simulink model "boost_simulink"  (R2021a)
settings: Solver=FixedStepDiscrete  StartTime=0.0  StopTime=0.5  FixedStep=sampleTime  MaxStep=1e-4  RelTol=1e-4  EnableMultiTasking=on
InitFcn:
  | boost_parameters
model workspace (MAT data in the model file):
  Phase1 = 0
values from neighbouring files (symbols this model uses):
  CoutModulesp = 271e-6    (= 0.000271)    [boost_parameters.m]    (also in unbalance_boost.m)
  CoutModuless = 544e-6    (= 0.000544)    [boost_parameters.m]
  D = (1-Vin/Vout)    (= 0.4)    [boost_parameters.m]    (also in calculations.m = (1-VinOneModule/VoutOneModule); flying_capacitor_parameters.m = 0.25; unbalance_boost.m = 0.25)
  Lcoilsp = 0.517e-3    (= 0.000517)    [boost_parameters.m]    (also in unbalance_boost.m = 0.001034)
  Lcoilss = 0.129e-3    (= 0.000129)    [boost_parameters.m]
  ModuleAPhase = 0    [boost_parameters.m]    (also in flying_capacitor_parameters.m = 90; unbalance_boost.m)
  ModuleBPhase = 180    [boost_parameters.m]    (also in flying_capacitor_parameters.m = 270; unbalance_boost.m = 90)
  ModuleCPhase = 180    [boost_parameters.m]    (also in flying_capacitor_parameters.m = 0)
  ModuleDPhase = 0    [boost_parameters.m]    (also in flying_capacitor_parameters.m = 180)
  Rcoil = 1e-3    (= 0.001)    [boost_parameters.m]    (also in unbalance_boost.m)
  sampleTime = 5e-8    (= 5e-08)    [boost_parameters.m]    (also in flying_capacitor_parameters.m = 5e-07; unbalance_boost.m)
  Vin = 900    [boost_parameters.m]    (also in flying_capacitor_parameters.m; main.m = 880; unbalance_boost.m)
libraries: spsSeriesRLCBranchLib x19, spsVoltageMeasurementLib x19, spsCurrentMeasurementLib x13, spsDiodeLib x8, spsIGBTDiodeLib x8, simulink x8, spsTriangleGeneratorLib x4, spsDCVoltageSourceLib x2, spspowerguiLib x1
settings Model: Creator=The MathWorks, Inc.  LastModifiedBy=enes_
settings SolverCC: AlgebraicLoopSolver=TrustRegion  SolverResetMethod=Robust
settings OptimizationCC: EfficientFloat2IntCast=on  LifeSpan=inf
settings DebuggingCC: ReadBeforeWriteMsg=DisableAll  WriteAfterWriteMsg=DisableAll  WriteAfterReadMsg=DisableAll  UniqueDataStoreMsg=error  StrictBusMsg=ErrorOnBusTreatedAsVector  SFUnexpectedBacktrackingDiag=warning  SFNoUnconditionalDefaultTransitionDiag=warning  SFExecutionAtInitializationDiag=none  SFMachineParentedDataDiag=warning  ArithmeticOperatorsInVariantConditions=warning
settings ModelReferenceCC: UpdateModelReferenceTargets=IfOutOfDate
settings SFSimCC: SFSimEcho=off  SimUseLocalCustomCode=off  CustomCodeUndefinedFunction=UseInterfaceOnly
settings RTWCC: RTWUseLocalCustomCode=off
settings CodeAppCC: StateflowObjectComments=on
settings GRTTargetCC: TargetLangStandard=C89/C90 (ANSI)
settings ConfigComp: CovMetricSettings=dw  CovSaveCumulativeToWorkspaceVar=on  CovSaveSingleToWorkspaceVar=on  CovExternalEMLEnable=off
settings SimscapeCC: SimscapeNormalizeSystem=off  SimscapeNominalValues={1, 'bar'; 1, 'cm^3/s'; 1, 'bar*kg/s'; 1, 'kJ/kg'; 1, 'kW'; }

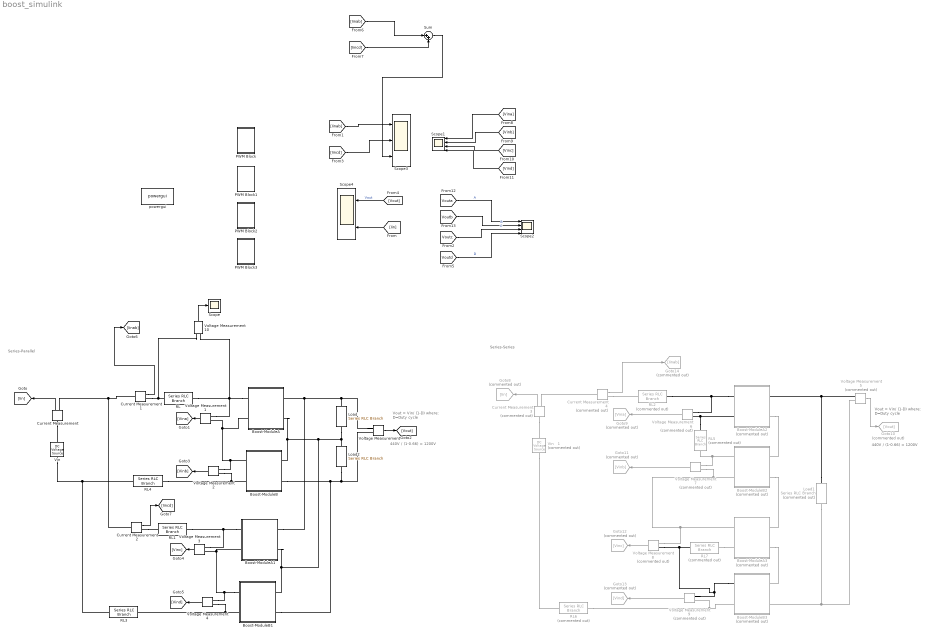
== system boost_simulink ==
  note: Series-Parallel
  note: Vout = Vin/ (1-D)
      | where: D=Duty cycle
  note: 440V / (1-0.66) = 1200V
  note: Series-Series
  note: 440V / (1-0.66) = 1200V
  note: Vout = Vin/ (1-D)
      | where: D=Duty cycle
  Boost-ModuleA : Subsystem
  Boost-ModuleA1 : Subsystem
  Boost-ModuleA2 : Subsystem  Commented=on
  Boost-ModuleA3 : Subsystem  Commented=on
  Boost-ModuleB : Subsystem
  Boost-ModuleB1 : Subsystem
  Boost-ModuleB2 : Subsystem  Commented=on
  Boost-ModuleB3 : Subsystem  Commented=on
  Current Measurement : spsCurrentMeasurementLib/Current Measurement  PhasorSimulation=off  OutputType=Complex  PSBequivalent=0
  Current Measurement1 : spsCurrentMeasurementLib/Current Measurement  PhasorSimulation=off  OutputType=Complex  PSBequivalent=0
  Current Measurement2 : spsCurrentMeasurementLib/Current Measurement  PhasorSimulation=off  OutputType=Complex  PSBequivalent=0
  Current Measurement3 : spsCurrentMeasurementLib/Current Measurement  Commented=on  PhasorSimulation=off  OutputType=Complex  PSBequivalent=0
  Current Measurement4 : spsCurrentMeasurementLib/Current Measurement  Commented=on  PhasorSimulation=off  OutputType=Complex  PSBequivalent=0
  Goto10 : Goto  Commented=on  GotoTag=Vout
  Goto11 : Goto  Commented=on  GotoTag=Vinb
  Goto12 : Goto  Commented=on  GotoTag=Vinc
  Goto13 : Goto  Commented=on  GotoTag=Vind
  Goto14 : Goto  Commented=on  GotoTag=Iinab
  Goto8 : Goto  Commented=on  GotoTag=Iin
  Goto9 : Goto  Commented=on  GotoTag=Vina
  Load : spsSeriesRLCBranchLib/Series RLC Branch  LConnTagsString=__new0  RConnTagsString=__new0  BranchType=R  Resistance=36  Inductance=200e-6  SetiL0=off  InitialCurrent=0  Capacitance=400e-6  Setx0=off  InitialVoltage=0  Measurements=None
  Load1 : spsSeriesRLCBranchLib/Series RLC Branch  Commented=on  LConnTagsString=__new0  RConnTagsString=__new0  BranchType=R  Resistance=72  Inductance=200e-6  SetiL0=off  InitialCurrent=0  Capacitance=400e-6  Setx0=off  InitialVoltage=0  Measurements=None
  Load2 : spsSeriesRLCBranchLib/Series RLC Branch  LConnTagsString=__new0  RConnTagsString=__new0  BranchType=R  Resistance=36  Inductance=200e-6  SetiL0=off  InitialCurrent=0  Capacitance=400e-6  Setx0=off  InitialVoltage=0  Measurements=None
  PWM Block : Subsystem
  PWM Block1 : Subsystem
  PWM Block2 : Subsystem
  PWM Block3 : Subsystem
  RL{,1,3..4} (4 alike) : spsSeriesRLCBranchLib/Series RLC Branch  LConnTagsString=__new0  RConnTagsString=__new0  BranchType=L  Resistance=Rcoil  Inductance=Lcoilsp  SetiL0=off  InitialCurrent=8  Capacitance=1e-6  Setx0=off  InitialVoltage=0  Measurements=None
  RL{2,5..7} (4 alike) : spsSeriesRLCBranchLib/Series RLC Branch  Commented=on  LConnTagsString=__new0  RConnTagsString=__new0  BranchType=L  Resistance=Rcoil  Inductance=Lcoilss  SetiL0=off  InitialCurrent=8  Capacitance=1e-6  Setx0=off  InitialVoltage=0  Measurements=None
  Scope : Scope
  Scope1 : Scope  NumInputPorts=4
  Scope2 : Scope  NumInputPorts=4
  Scope3 : Scope  NumInputPorts=3
  Scope4 : Scope  NumInputPorts=2
  Sum : Sum  Inputs=|++
  "Vin   " : spsDCVoltageSourceLib/DC Voltage Source  Amplitude=Vin  Measurements=None
  Vin   1 : spsDCVoltageSourceLib/DC Voltage Source  Commented=on  Amplitude=Vin  Measurements=None
  Voltage Measurement{,1..4,10} (6 alike) : spsVoltageMeasurementLib/Voltage Measurement  PhasorSimulation=off  OutputType=Complex  PSBequivalent=0
  Voltage Measurement{5..9} (5 alike) : spsVoltageMeasurementLib/Voltage Measurement  Commented=on  PhasorSimulation=off  OutputType=Complex  PSBequivalent=0
  powergui : spspowerguiLib/powergui  Priority=1  SimulationMode=Discrete  SampleTime=sampleTime  frequency=60  Iterations=50  frequencyindice=0  Pbase=100e6  ErrMax=1e-4  UnitsV=kV  UnitsW=MW  buscounter=0  FunctionMessages=off  echomessages=off  EnableUseOfTLC=off  CurrentSourceSwitches=off  DisableSnubberDevices=off  DisableRonSwitches=off  DisableVfSwitches=off  DisplayEquations=off  AutomaticDiscreteSolvers=off  SolverType=Tustin/Backward Euler (TBE)  Interpol=off  ExternalGateDelay=off  methode=off  Ts=100  x0status=blocks  SPID=on  SwTol=0  HookPort=off  NonlinearTolerance=1e-4  nMaxIteration=100  ContinueOnMaxIteration=off  RestoreLinks=warning  ResistiveCurrentMeasurement=off  Frange=[0:2:500]  Ylog=off  Xlog=on  ShowGrid=off  save=off  variable=ZData  structure=0  ZoomFFT=off  StartTime=0.0  cycles=1  DisplayStyle=1  fundamental=60  FreqAxis=off  MaxFrequency=1000  frequencyindicesteady=1  RmsSteady=1  display=off
  wires:
  [Vout] -> Scope4/1  "Vout"
  [Iin] -> Scope4/2
  [Vina] -> Scope1/1
  [Vinb] -> Scope1/2
  [Vinc] -> Scope1/3
  [Vind] -> Scope1/4
  [Iincd] -> Scope3/2
  [Iinab] -> Scope3/1
  [Vouta] -> Scope2/1  "A"
  [Voutb] -> Scope2/2  "B"
  [Voutc] -> Scope2/3  "C"
  [Voutd] -> Scope2/4  "D"
  Current Measurement2/1 -> [Iincd]
  Current Measurement1/1 -> [Iinab]
  Voltage Measurement2/1 -> [Vinb]
  Voltage Measurement4/1 -> [Vind]
  Voltage Measurement3/1 -> [Vinc]
  Voltage Measurement1/1 -> [Vina]
  Current Measurement/1 -> [Iin]
  Voltage Measurement/1 -> [Vout]
  Current Measurement4/1 -> Goto14/1
  Voltage Measurement7/1 -> Goto11/1
  Voltage Measurement9/1 -> Goto13/1
  Voltage Measurement8/1 -> Goto12/1
  Current Measurement3/1 -> Goto8/1
  Voltage Measurement5/1 -> Goto10/1
  Voltage Measurement6/1 -> Goto9/1
  [Iincd] -> Sum/2
  [Iinab] -> Sum/1
  Sum/1 -> Scope3/3
  Voltage Measurement10/1 -> Scope/1
  connections:
  Current Measurement2/RConn1 -- RL1/LConn1
  Current Measurement1/RConn1 -- Voltage Measurement10/LConn1 -- RL/LConn1
  Boost-ModuleA/LConn1 -- RL/RConn1 -- Voltage Measurement10/LConn2 -- Voltage Measurement1/LConn1
  Boost-ModuleA1/LConn1 -- RL1/RConn1 -- Voltage Measurement3/LConn1
  Current Measurement1/LConn1 -- Current Measurement2/LConn1 -- Current Measurement/RConn1
  Boost-ModuleB/RConn2 -- Boost-ModuleB1/RConn2 -- Load2/RConn1 -- Voltage Measurement/LConn2
  Boost-ModuleA/LConn2 -- Voltage Measurement2/LConn1 -- Boost-ModuleB/LConn1 -- Voltage Measurement1/LConn2
  Boost-ModuleB1/LConn1 -- Boost-ModuleA1/LConn2 -- Voltage Measurement3/LConn2 -- Voltage Measurement4/LConn1
  Voltage Measurement2/LConn2 -- RL4/RConn1 -- Boost-ModuleB/LConn2
  Voltage Measurement/LConn1 -- Load/LConn1 -- Boost-ModuleA1/RConn1 -- Boost-ModuleA/RConn1
  Current Measurement/LConn1 -- "Vin   "/RConn1
  RL5/LConn1 -- Boost-ModuleA2/LConn2 -- Voltage Measurement6/LConn2
  Boost-ModuleA2/LConn1 -- RL2/RConn1 -- Voltage Measurement6/LConn1
  Load1/RConn1 -- Voltage Measurement5/LConn2 -- Boost-ModuleB3/RConn2
  Boost-ModuleB2/LConn2 -- Voltage Measurement7/LConn2 -- Boost-ModuleA3/LConn1 -- Voltage Measurement8/LConn1
  Current Measurement4/LConn1 -- Current Measurement3/RConn1
  Boost-ModuleB3/LConn1 -- RL7/LConn1 -- Voltage Measurement8/LConn2 -- Voltage Measurement9/LConn1
  Load1/LConn1 -- Voltage Measurement5/LConn1 -- Boost-ModuleA2/RConn1
  Boost-ModuleA2/RConn2 -- Boost-ModuleB2/RConn1
  Current Measurement3/LConn1 -- Vin   1/RConn1
  Current Measurement4/RConn1 -- RL2/LConn1
  Boost-ModuleA3/RConn2 -- Boost-ModuleB3/RConn1
  Boost-ModuleB3/LConn2 -- RL6/RConn1 -- Voltage Measurement9/LConn2
  Boost-ModuleB2/RConn2 -- Boost-ModuleA3/RConn1
  Boost-ModuleB1/LConn2 -- Voltage Measurement4/LConn2 -- RL3/RConn1
  RL3/LConn1 -- "Vin   "/LConn1 -- RL4/LConn1
  RL5/RConn1 -- Boost-ModuleB2/LConn1 -- Voltage Measurement7/LConn1
  Vin   1/LConn1 -- RL6/LConn1
  RL7/RConn1 -- Boost-ModuleA3/LConn2
  Boost-ModuleA1/RConn2 -- Boost-ModuleB/RConn1 -- Boost-ModuleA/RConn2 -- Load/RConn1 -- Load2/LConn1 -- Boost-ModuleB1/RConn1

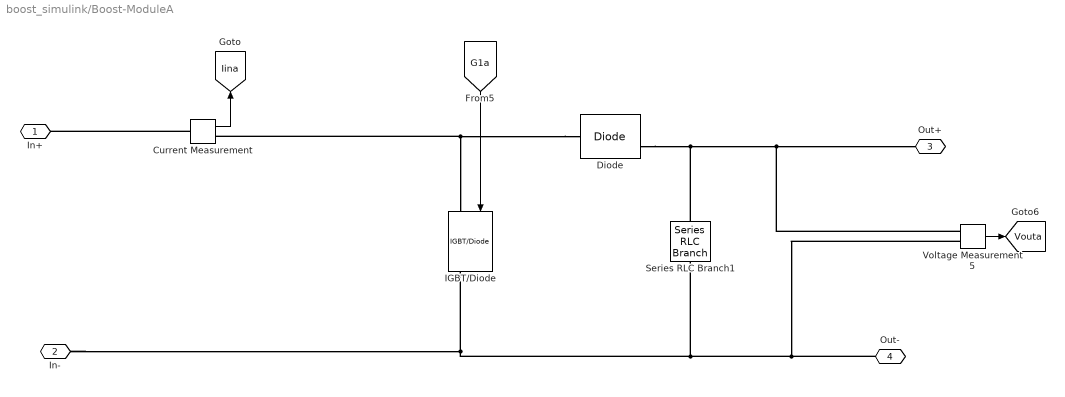
== system boost_simulink/Boost-ModuleA ==
  Current Measurement : spsCurrentMeasurementLib/Current Measurement  PhasorSimulation=off  OutputType=Complex  PSBequivalent=0
  Diode : spsDiodeLib/Diode  Ron=0.001  Lon=0  Vf=0.8  IC=0  UseSnubber=0  Rs=500  Cs=250e-9  Measurements=on
  IGBT/Diode : spsIGBTDiodeLib/IGBT//Diode  Ron=1e-3  Rs=1e5  Cs=inf  Measurements=on
  Series RLC Branch1 : spsSeriesRLCBranchLib/Series RLC Branch  LConnTagsString=__new0  RConnTagsString=__new0  BranchType=C  Resistance=1e-4  Inductance=200e-6  SetiL0=off  InitialCurrent=0  Capacitance=CoutModulesp  Setx0=off  InitialVoltage=1200  Measurements=None
  Voltage Measurement5 : spsVoltageMeasurementLib/Voltage Measurement  PhasorSimulation=off  OutputType=Complex  PSBequivalent=0
  In+ : PMIOPort  Side=Left
  In- : PMIOPort  Port=2  Side=Left
  Out+ : PMIOPort  Port=3  Side=Right
  Out- : PMIOPort  Port=4  Side=Right
  tag scope: Iina=global, Vouta=global
  wires:
  [G1a] -> IGBT/Diode/1
  Current Measurement/1 -> [Iina]
  Voltage Measurement5/1 -> [Vouta]
  connections:
  Diode/LConn1 -- IGBT/Diode/LConn1 -- Current Measurement/RConn1
  Series RLC Branch1/LConn1 -- Diode/RConn1 -- Voltage Measurement5/LConn1 -- Out+/RConn1
  Current Measurement/LConn1 -- In+/RConn1
  Out-/RConn1 -- Voltage Measurement5/LConn2 -- In-/RConn1 -- IGBT/Diode/RConn1 -- Series RLC Branch1/RConn1

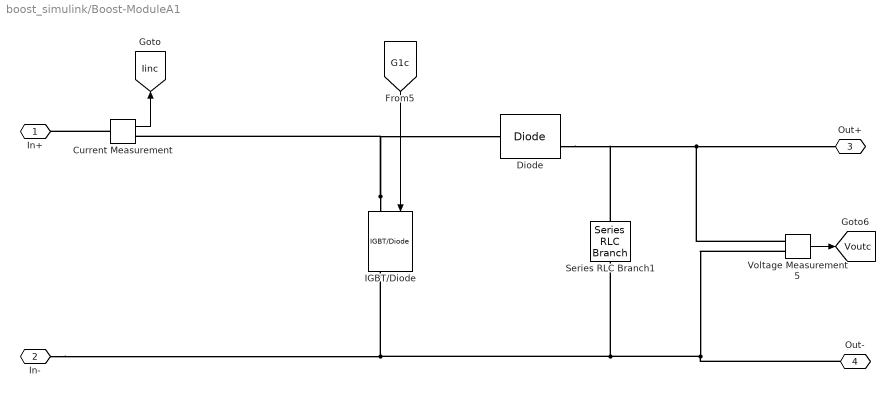
== system boost_simulink/Boost-ModuleA1 ==
  Current Measurement : spsCurrentMeasurementLib/Current Measurement  PhasorSimulation=off  OutputType=Complex  PSBequivalent=0
  Diode : spsDiodeLib/Diode  Ron=0.001  Lon=0  Vf=0.8  IC=0  UseSnubber=0  Rs=500  Cs=250e-9  Measurements=on
  IGBT/Diode : spsIGBTDiodeLib/IGBT//Diode  Ron=1e-3  Rs=1e5  Cs=inf  Measurements=on
  Series RLC Branch1 : spsSeriesRLCBranchLib/Series RLC Branch  LConnTagsString=__new0  RConnTagsString=__new0  BranchType=C  Resistance=1e-4  Inductance=200e-6  SetiL0=off  InitialCurrent=0  Capacitance=CoutModulesp  Setx0=off  InitialVoltage=1200  Measurements=None
  Voltage Measurement5 : spsVoltageMeasurementLib/Voltage Measurement  PhasorSimulation=off  OutputType=Complex  PSBequivalent=0
  In+ : PMIOPort  Side=Left
  In- : PMIOPort  Port=2  Side=Left
  Out+ : PMIOPort  Port=3  Side=Right
  Out- : PMIOPort  Port=4  Side=Right
  tag scope: Iinc=global, Voutc=global
  wires:
  [G1c] -> IGBT/Diode/1
  Current Measurement/1 -> [Iinc]
  Voltage Measurement5/1 -> [Voutc]
  connections:
  IGBT/Diode/LConn1 -- Diode/LConn1 -- Current Measurement/RConn1
  Voltage Measurement5/LConn1 -- Out+/RConn1 -- Series RLC Branch1/LConn1 -- Diode/RConn1
  Current Measurement/LConn1 -- In+/RConn1
  Voltage Measurement5/LConn2 -- Out-/RConn1 -- Series RLC Branch1/RConn1 -- In-/RConn1 -- IGBT/Diode/RConn1

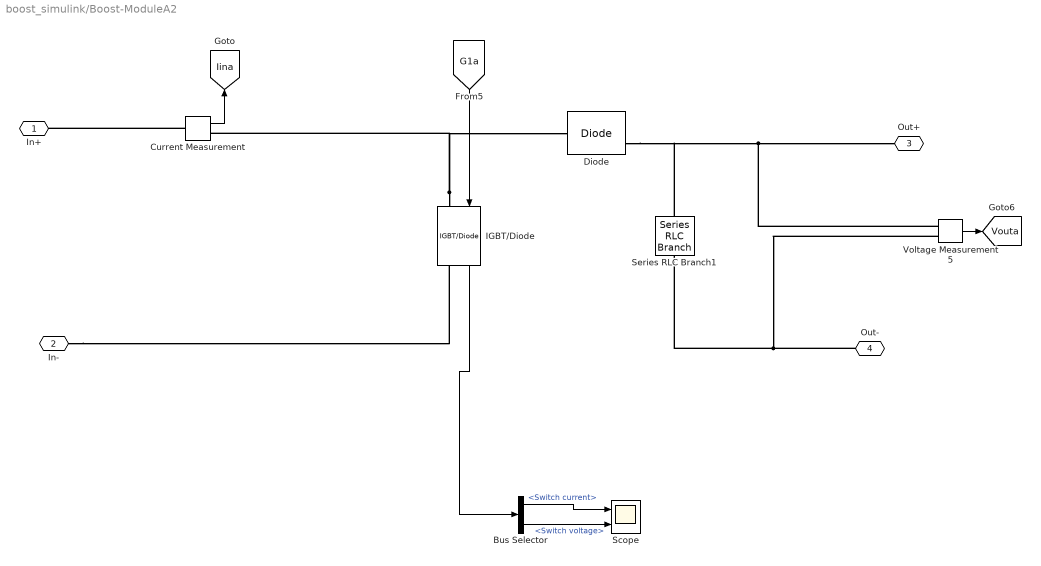
== system boost_simulink/Boost-ModuleA2 ==
  Bus Selector : BusSelector  OutputSignals=Switch current,Switch voltage
  Current Measurement : spsCurrentMeasurementLib/Current Measurement  PhasorSimulation=off  OutputType=Complex  PSBequivalent=0
  Diode : spsDiodeLib/Diode  Ron=0.001  Lon=0  Vf=0.8  IC=0  UseSnubber=0  Rs=500  Cs=250e-9  Measurements=on
  IGBT/Diode : spsIGBTDiodeLib/IGBT//Diode  Ron=1e-3  Rs=1e5  Cs=inf  Measurements=on
  Scope : Scope  NumInputPorts=2
  Series RLC Branch1 : spsSeriesRLCBranchLib/Series RLC Branch  LConnTagsString=__new0  RConnTagsString=__new0  BranchType=C  Resistance=1e-4  Inductance=200e-6  SetiL0=off  InitialCurrent=0  Capacitance=CoutModuless  Setx0=off  InitialVoltage=1200  Measurements=None
  Voltage Measurement5 : spsVoltageMeasurementLib/Voltage Measurement  PhasorSimulation=off  OutputType=Complex  PSBequivalent=0
  In+ : PMIOPort  Side=Left
  In- : PMIOPort  Port=2  Side=Left
  Out+ : PMIOPort  Port=3  Side=Right
  Out- : PMIOPort  Port=4  Side=Right
  tag scope: Iina=global, Vouta=global
  wires:
  [G1a] -> IGBT/Diode/1
  Current Measurement/1 -> [Iina]
  Voltage Measurement5/1 -> [Vouta]
  IGBT/Diode/1 -> Bus Selector/1
  Bus Selector/1 -> Scope/1  "<Switch current>"
  Bus Selector/2 -> Scope/2  "<Switch voltage>"
  connections:
  IGBT/Diode/LConn1 -- Diode/LConn1 -- Current Measurement/RConn1
  Voltage Measurement5/LConn1 -- Out+/RConn1 -- Series RLC Branch1/LConn1 -- Diode/RConn1
  Current Measurement/LConn1 -- In+/RConn1
  In-/RConn1 -- IGBT/Diode/RConn1
  Out-/RConn1 -- Series RLC Branch1/RConn1 -- Voltage Measurement5/LConn2

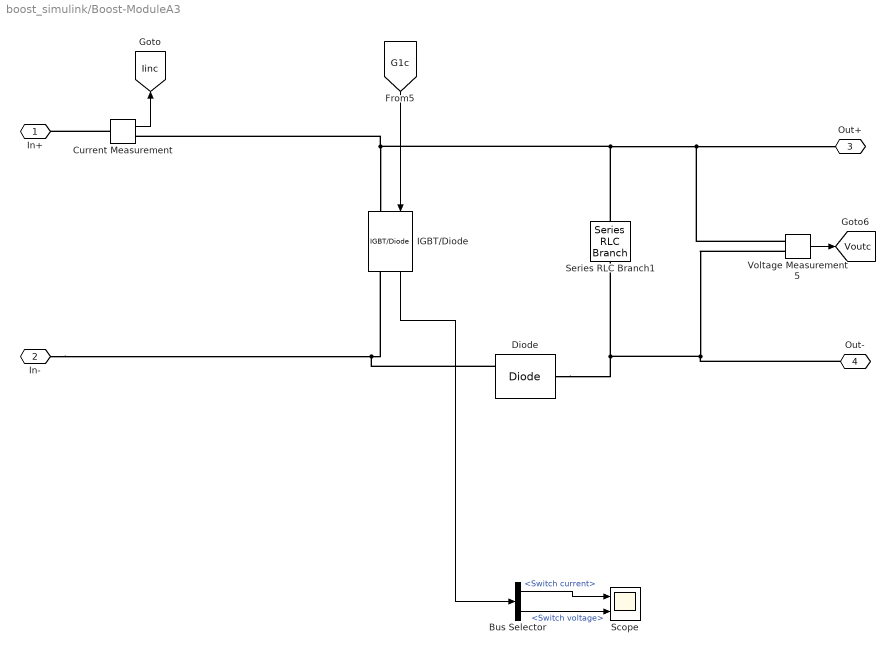
== system boost_simulink/Boost-ModuleA3 ==
  Bus Selector : BusSelector  OutputSignals=Switch current,Switch voltage
  Current Measurement : spsCurrentMeasurementLib/Current Measurement  PhasorSimulation=off  OutputType=Complex  PSBequivalent=0
  Diode : spsDiodeLib/Diode  Ron=0.001  Lon=0  Vf=0.8  IC=0  UseSnubber=0  Rs=500  Cs=250e-9  Measurements=on
  IGBT/Diode : spsIGBTDiodeLib/IGBT//Diode  Ron=1e-3  Rs=1e5  Cs=inf  Measurements=on
  Scope : Scope  NumInputPorts=2
  Series RLC Branch1 : spsSeriesRLCBranchLib/Series RLC Branch  LConnTagsString=__new0  RConnTagsString=__new0  BranchType=C  Resistance=1e-4  Inductance=200e-6  SetiL0=off  InitialCurrent=0  Capacitance=CoutModuless  Setx0=off  InitialVoltage=1200  Measurements=None
  Voltage Measurement5 : spsVoltageMeasurementLib/Voltage Measurement  PhasorSimulation=off  OutputType=Complex  PSBequivalent=0
  In+ : PMIOPort  Side=Left
  In- : PMIOPort  Port=2  Side=Left
  Out+ : PMIOPort  Port=3  Side=Right
  Out- : PMIOPort  Port=4  Side=Right
  tag scope: Iinc=global, Voutc=global
  wires:
  [G1c] -> IGBT/Diode/1
  Current Measurement/1 -> [Iinc]
  Voltage Measurement5/1 -> [Voutc]
  IGBT/Diode/1 -> Bus Selector/1
  Bus Selector/1 -> Scope/1  "<Switch current>"
  Bus Selector/2 -> Scope/2  "<Switch voltage>"
  connections:
  Voltage Measurement5/LConn1 -- Out+/RConn1 -- Current Measurement/RConn1 -- IGBT/Diode/LConn1 -- Series RLC Branch1/LConn1
  Current Measurement/LConn1 -- In+/RConn1
  Voltage Measurement5/LConn2 -- Out-/RConn1 -- Series RLC Branch1/RConn1 -- Diode/LConn1
  In-/RConn1 -- Diode/RConn1 -- IGBT/Diode/RConn1

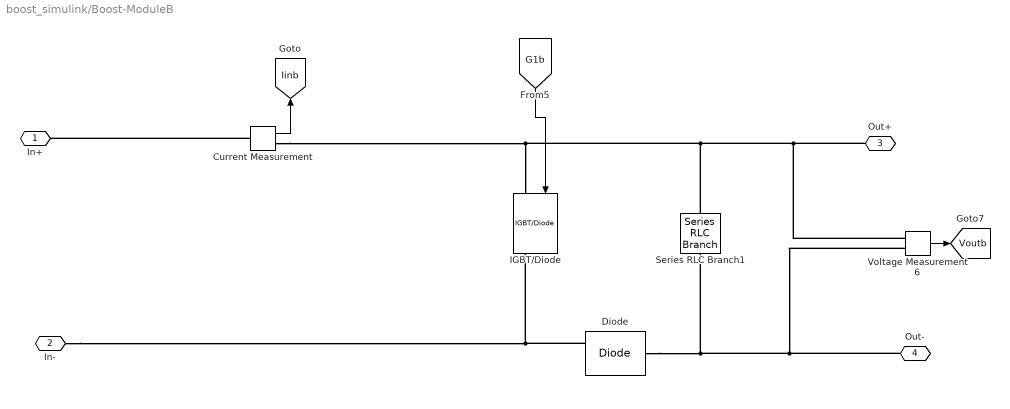
== system boost_simulink/Boost-ModuleB ==
  Current Measurement : spsCurrentMeasurementLib/Current Measurement  PhasorSimulation=off  OutputType=Complex  PSBequivalent=0
  Diode : spsDiodeLib/Diode  Ron=0.001  Lon=0  Vf=0.8  IC=0  UseSnubber=0  Rs=500  Cs=250e-9  Measurements=on
  IGBT/Diode : spsIGBTDiodeLib/IGBT//Diode  Ron=1e-3  Rs=1e5  Cs=inf  Measurements=on
  Series RLC Branch1 : spsSeriesRLCBranchLib/Series RLC Branch  LConnTagsString=__new0  RConnTagsString=__new0  BranchType=C  Resistance=1e-4  Inductance=200e-6  SetiL0=off  InitialCurrent=0  Capacitance=CoutModulesp  Setx0=off  InitialVoltage=1200  Measurements=None
  Voltage Measurement6 : spsVoltageMeasurementLib/Voltage Measurement  PhasorSimulation=off  OutputType=Complex  PSBequivalent=0
  In+ : PMIOPort  Side=Left
  In- : PMIOPort  Port=2  Side=Left
  Out+ : PMIOPort  Port=3  Side=Right
  Out- : PMIOPort  Port=4  Side=Right
  tag scope: Iinb=global, Voutb=global
  wires:
  Current Measurement/1 -> [Iinb]
  [G1b] -> IGBT/Diode/1
  Voltage Measurement6/1 -> [Voutb]
  connections:
  Out+/RConn1 -- Voltage Measurement6/LConn1 -- Series RLC Branch1/LConn1 -- Current Measurement/RConn1 -- IGBT/Diode/LConn1
  Out-/RConn1 -- Voltage Measurement6/LConn2 -- Diode/LConn1 -- Series RLC Branch1/RConn1
  Current Measurement/LConn1 -- In+/RConn1
  In-/RConn1 -- Diode/RConn1 -- IGBT/Diode/RConn1

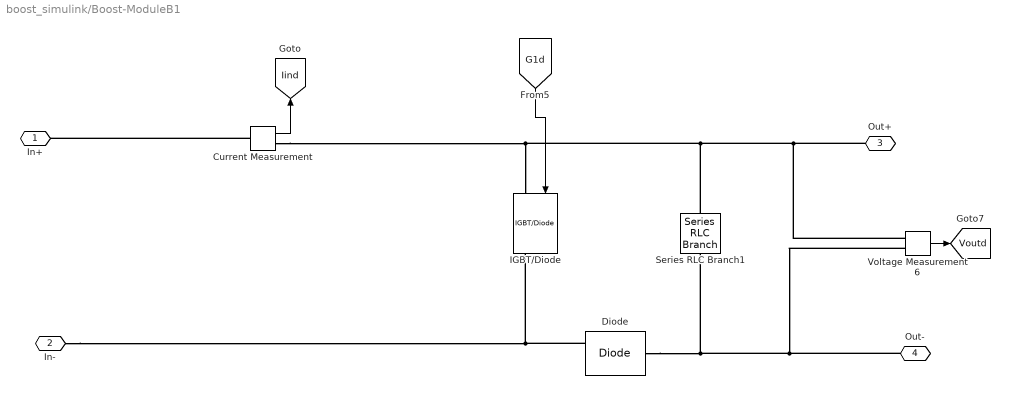
== system boost_simulink/Boost-ModuleB1 ==
  Current Measurement : spsCurrentMeasurementLib/Current Measurement  PhasorSimulation=off  OutputType=Complex  PSBequivalent=0
  Diode : spsDiodeLib/Diode  Ron=0.001  Lon=0  Vf=0.8  IC=0  UseSnubber=0  Rs=500  Cs=250e-9  Measurements=on
  IGBT/Diode : spsIGBTDiodeLib/IGBT//Diode  Ron=1e-3  Rs=1e5  Cs=inf  Measurements=on
  Series RLC Branch1 : spsSeriesRLCBranchLib/Series RLC Branch  LConnTagsString=__new0  RConnTagsString=__new0  BranchType=C  Resistance=1e-4  Inductance=200e-6  SetiL0=off  InitialCurrent=0  Capacitance=CoutModulesp  Setx0=off  InitialVoltage=1200  Measurements=None
  Voltage Measurement6 : spsVoltageMeasurementLib/Voltage Measurement  PhasorSimulation=off  OutputType=Complex  PSBequivalent=0
  In+ : PMIOPort  Side=Left
  In- : PMIOPort  Port=2  Side=Left
  Out+ : PMIOPort  Port=3  Side=Right
  Out- : PMIOPort  Port=4  Side=Right
  tag scope: Iind=global, Voutd=global
  wires:
  Current Measurement/1 -> [Iind]
  [G1d] -> IGBT/Diode/1
  Voltage Measurement6/1 -> [Voutd]
  connections:
  Current Measurement/RConn1 -- IGBT/Diode/LConn1 -- Series RLC Branch1/LConn1 -- Voltage Measurement6/LConn1 -- Out+/RConn1
  Diode/LConn1 -- Series RLC Branch1/RConn1 -- Out-/RConn1 -- Voltage Measurement6/LConn2
  Current Measurement/LConn1 -- In+/RConn1
  In-/RConn1 -- IGBT/Diode/RConn1 -- Diode/RConn1

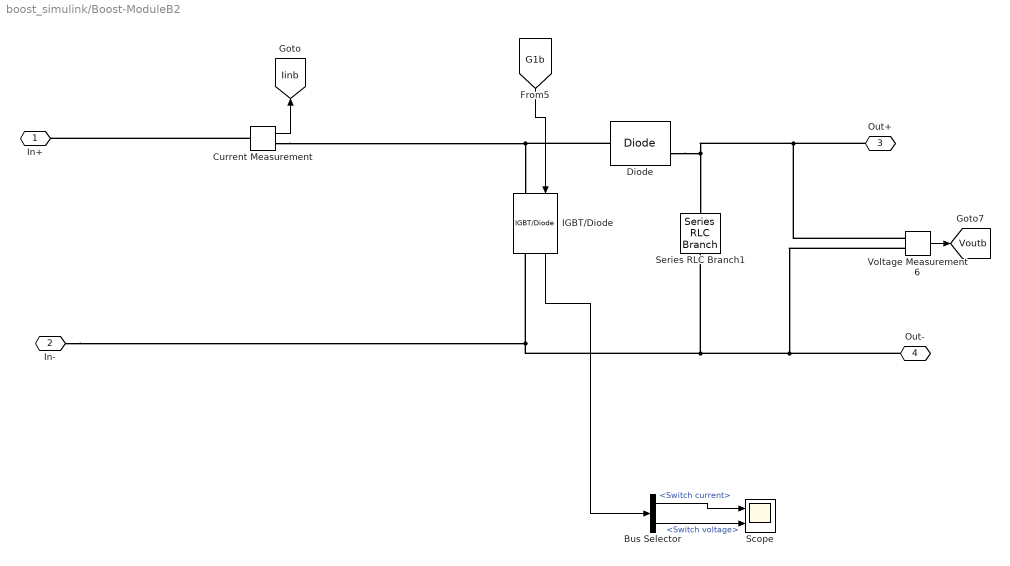
== system boost_simulink/Boost-ModuleB2 ==
  Bus Selector : BusSelector  OutputSignals=Switch current,Switch voltage
  Current Measurement : spsCurrentMeasurementLib/Current Measurement  PhasorSimulation=off  OutputType=Complex  PSBequivalent=0
  Diode : spsDiodeLib/Diode  Ron=0.001  Lon=0  Vf=0.8  IC=0  UseSnubber=0  Rs=500  Cs=250e-9  Measurements=on
  IGBT/Diode : spsIGBTDiodeLib/IGBT//Diode  Ron=1e-3  Rs=1e5  Cs=inf  Measurements=on
  Scope : Scope  NumInputPorts=2
  Series RLC Branch1 : spsSeriesRLCBranchLib/Series RLC Branch  LConnTagsString=__new0  RConnTagsString=__new0  BranchType=C  Resistance=1e-4  Inductance=200e-6  SetiL0=off  InitialCurrent=0  Capacitance=CoutModuless  Setx0=off  InitialVoltage=1200  Measurements=None
  Voltage Measurement6 : spsVoltageMeasurementLib/Voltage Measurement  PhasorSimulation=off  OutputType=Complex  PSBequivalent=0
  In+ : PMIOPort  Side=Left
  In- : PMIOPort  Port=2  Side=Left
  Out+ : PMIOPort  Port=3  Side=Right
  Out- : PMIOPort  Port=4  Side=Right
  tag scope: Iinb=global, Voutb=global
  wires:
  Current Measurement/1 -> [Iinb]
  [G1b] -> IGBT/Diode/1
  Voltage Measurement6/1 -> [Voutb]
  IGBT/Diode/1 -> Bus Selector/1
  Bus Selector/1 -> Scope/1  "<Switch current>"
  Bus Selector/2 -> Scope/2  "<Switch voltage>"
  connections:
  Voltage Measurement6/LConn1 -- Out+/RConn1 -- Diode/RConn1 -- Series RLC Branch1/LConn1
  Current Measurement/LConn1 -- In+/RConn1
  Out-/RConn1 -- In-/RConn1 -- IGBT/Diode/RConn1 -- Series RLC Branch1/RConn1 -- Voltage Measurement6/LConn2
  Current Measurement/RConn1 -- IGBT/Diode/LConn1 -- Diode/LConn1

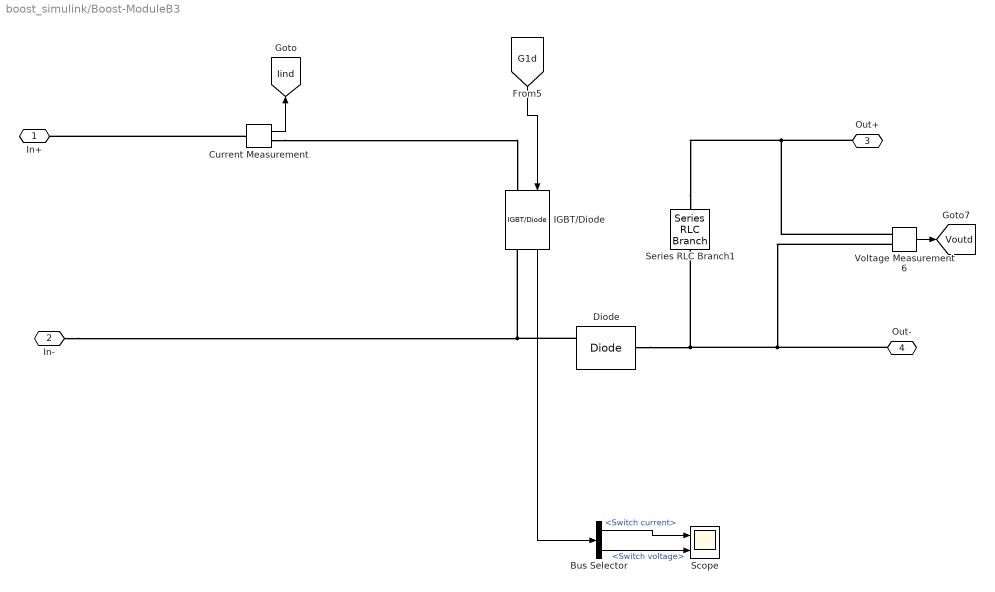
== system boost_simulink/Boost-ModuleB3 ==
  Bus Selector : BusSelector  OutputSignals=Switch current,Switch voltage
  Current Measurement : spsCurrentMeasurementLib/Current Measurement  PhasorSimulation=off  OutputType=Complex  PSBequivalent=0
  Diode : spsDiodeLib/Diode  Ron=0.001  Lon=0  Vf=0.8  IC=0  UseSnubber=0  Rs=500  Cs=250e-9  Measurements=on
  IGBT/Diode : spsIGBTDiodeLib/IGBT//Diode  Ron=1e-3  Rs=1e5  Cs=inf  Measurements=on
  Scope : Scope  NumInputPorts=2
  Series RLC Branch1 : spsSeriesRLCBranchLib/Series RLC Branch  LConnTagsString=__new0  RConnTagsString=__new0  BranchType=C  Resistance=1e-4  Inductance=200e-6  SetiL0=off  InitialCurrent=0  Capacitance=CoutModuless  Setx0=off  InitialVoltage=1200  Measurements=None
  Voltage Measurement6 : spsVoltageMeasurementLib/Voltage Measurement  PhasorSimulation=off  OutputType=Complex  PSBequivalent=0
  In+ : PMIOPort  Side=Left
  In- : PMIOPort  Port=2  Side=Left
  Out+ : PMIOPort  Port=3  Side=Right
  Out- : PMIOPort  Port=4  Side=Right
  tag scope: Iind=global, Voutd=global
  wires:
  Current Measurement/1 -> [Iind]
  [G1d] -> IGBT/Diode/1
  Voltage Measurement6/1 -> [Voutd]
  IGBT/Diode/1 -> Bus Selector/1
  Bus Selector/1 -> Scope/1  "<Switch current>"
  Bus Selector/2 -> Scope/2  "<Switch voltage>"
  connections:
  Series RLC Branch1/LConn1 -- Voltage Measurement6/LConn1 -- Out+/RConn1
  Diode/LConn1 -- Series RLC Branch1/RConn1 -- Out-/RConn1 -- Voltage Measurement6/LConn2
  Current Measurement/LConn1 -- In+/RConn1
  In-/RConn1 -- IGBT/Diode/RConn1 -- Diode/RConn1
  Current Measurement/RConn1 -- IGBT/Diode/LConn1

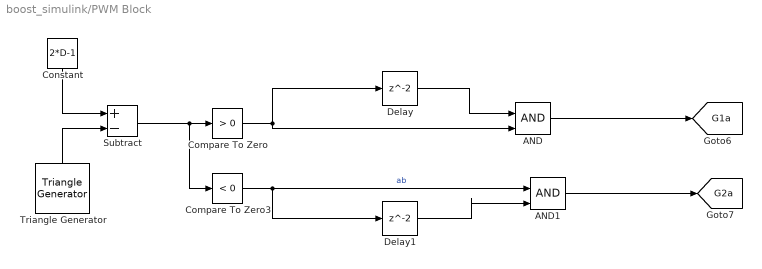
== system boost_simulink/PWM Block ==
  AND : Logic  IconShape=distinctive  AllPortsSameDT=off  OutDataTypeStr=boolean
  AND1 : Logic  IconShape=distinctive  AllPortsSameDT=off  OutDataTypeStr=boolean
  Compare To Zero : simulink/Logic and Bit Operations/Compare To Zero  relop=>  OutDataTypeStr=boolean
  Compare To Zero3 : simulink/Logic and Bit Operations/Compare To Zero  relop=<  OutDataTypeStr=boolean
  Constant : Constant  Value=2*D-1
  Delay : Delay
  Delay1 : Delay
  Subtract : Sum  Inputs=+-
  Triangle Generator : spsTriangleGeneratorLib/Triangle Generator  Freq=fsw  Phase=ModuleAPhase  Ts=sampleTime
  tag scope: G1a=global, G2a=global
  wires:
  Constant/1 -> Subtract/1
  Triangle Generator/1 -> Subtract/2
  Subtract/1 -> Compare To Zero3/1, Compare To Zero/1
  AND/1 -> [G1a]
  Compare To Zero/1 -> Delay/1, AND/2
  Delay/1 -> AND/1
  Compare To Zero3/1 -> Delay1/1, AND1/1  "ab"
  AND1/1 -> [G2a]
  Delay1/1 -> AND1/2

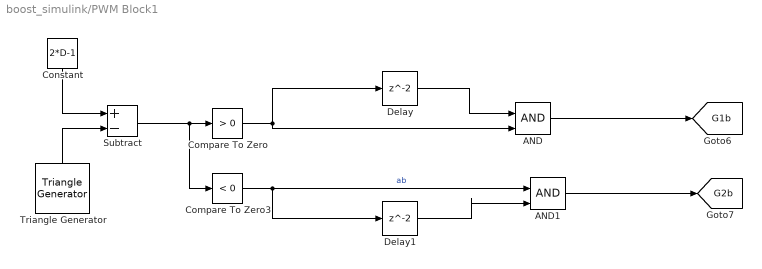
== system boost_simulink/PWM Block1 ==
  AND : Logic  IconShape=distinctive  AllPortsSameDT=off  OutDataTypeStr=boolean
  AND1 : Logic  IconShape=distinctive  AllPortsSameDT=off  OutDataTypeStr=boolean
  Compare To Zero : simulink/Logic and Bit Operations/Compare To Zero  relop=>  OutDataTypeStr=boolean
  Compare To Zero3 : simulink/Logic and Bit Operations/Compare To Zero  relop=<  OutDataTypeStr=boolean
  Constant : Constant  Value=2*D-1
  Delay : Delay
  Delay1 : Delay
  Subtract : Sum  Inputs=+-
  Triangle Generator : spsTriangleGeneratorLib/Triangle Generator  Freq=fsw  Phase=ModuleBPhase  Ts=sampleTime
  tag scope: G1b=global, G2b=global
  wires:
  Constant/1 -> Subtract/1
  Triangle Generator/1 -> Subtract/2
  Subtract/1 -> Compare To Zero3/1, Compare To Zero/1
  AND/1 -> [G1b]
  Compare To Zero/1 -> Delay/1, AND/2
  Delay/1 -> AND/1
  Compare To Zero3/1 -> Delay1/1, AND1/1  "ab"
  AND1/1 -> [G2b]
  Delay1/1 -> AND1/2

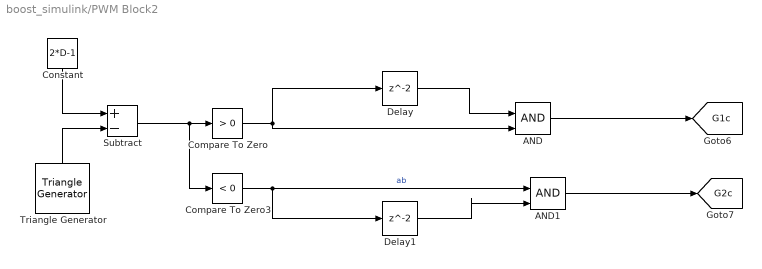
== system boost_simulink/PWM Block2 ==
  AND : Logic  IconShape=distinctive  AllPortsSameDT=off  OutDataTypeStr=boolean
  AND1 : Logic  IconShape=distinctive  AllPortsSameDT=off  OutDataTypeStr=boolean
  Compare To Zero : simulink/Logic and Bit Operations/Compare To Zero  relop=>  OutDataTypeStr=boolean
  Compare To Zero3 : simulink/Logic and Bit Operations/Compare To Zero  relop=<  OutDataTypeStr=boolean
  Constant : Constant  Value=2*D-1
  Delay : Delay
  Delay1 : Delay
  Subtract : Sum  Inputs=+-
  Triangle Generator : spsTriangleGeneratorLib/Triangle Generator  Freq=fsw  Phase=ModuleCPhase  Ts=sampleTime
  tag scope: G1c=global, G2c=global
  wires:
  Constant/1 -> Subtract/1
  Triangle Generator/1 -> Subtract/2
  Subtract/1 -> Compare To Zero3/1, Compare To Zero/1
  AND/1 -> [G1c]
  Compare To Zero/1 -> Delay/1, AND/2
  Delay/1 -> AND/1
  Compare To Zero3/1 -> Delay1/1, AND1/1  "ab"
  AND1/1 -> [G2c]
  Delay1/1 -> AND1/2

== system boost_simulink/PWM Block3 ==
  AND : Logic  IconShape=distinctive  AllPortsSameDT=off  OutDataTypeStr=boolean
  AND1 : Logic  IconShape=distinctive  AllPortsSameDT=off  OutDataTypeStr=boolean
  Compare To Zero : simulink/Logic and Bit Operations/Compare To Zero  relop=>  OutDataTypeStr=boolean
  Compare To Zero3 : simulink/Logic and Bit Operations/Compare To Zero  relop=<  OutDataTypeStr=boolean
  Constant : Constant  Value=2*D-1
  Delay : Delay
  Delay1 : Delay
  Subtract : Sum  Inputs=+-
  Triangle Generator : spsTriangleGeneratorLib/Triangle Generator  Freq=fsw  Phase=ModuleDPhase  Ts=sampleTime
  tag scope: G1d=global, G2d=global
  wires:
  Constant/1 -> Subtract/1
  Triangle Generator/1 -> Subtract/2
  Subtract/1 -> Compare To Zero3/1, Compare To Zero/1
  AND/1 -> [G1d]
  Compare To Zero/1 -> Delay/1, AND/2
  Delay/1 -> AND/1
  Compare To Zero3/1 -> Delay1/1, AND1/1  "ab"
  AND1/1 -> [G2d]
  Delay1/1 -> AND1/2
